simulink model "lab1_1"  (R2021b)
settings: Solver=VariableStepAuto  StartTime=0.0  StopTime=30  RelTol=10e-10  AbsTol=10e-10
values from neighbouring files (symbols this model uses):
  den = cell2mat(den)    [lab1.m]
  den1 = cell2mat(den1)    [lab1.m]
  num = cell2mat(num)    [lab1.m]
  num1 = cell2mat(num1)    [lab1.m]
settings Model: Creator=zhangshaoyang  LastModifiedBy=zhangshaoyang

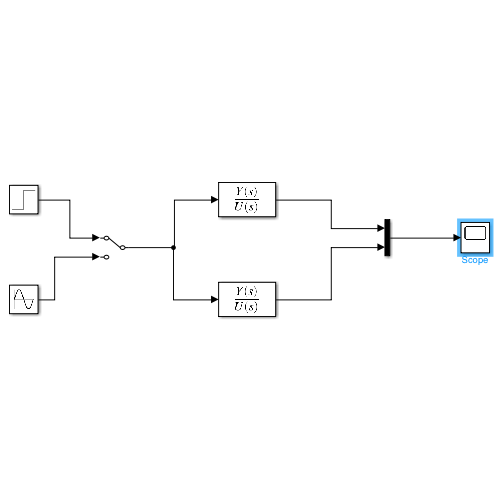
[thumbnail: Simulink's stored preview of the top-level diagram]
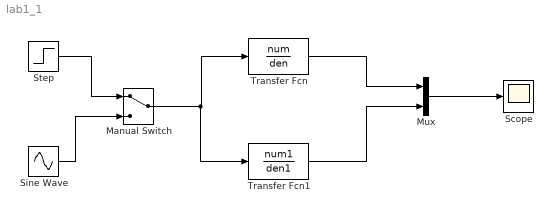
== system lab1_1 ==
  Manual Switch : ManualSwitch
  Mux : Mux  Inputs=2
  Scope : Scope
  Sine Wave : Sin  SampleTime=0
  Step : Step  SampleTime=0
  Transfer Fcn : TransferFcn  Numerator=num  Denominator=den
  Transfer Fcn1 : TransferFcn  Numerator=num1  Denominator=den1
  wires:
  Step/1 -> Manual Switch/1
  Sine Wave/1 -> Manual Switch/2
  Manual Switch/1 -> Transfer Fcn1/1, Transfer Fcn/1
  Transfer Fcn/1 -> Mux/1
  Transfer Fcn1/1 -> Mux/2
  Mux/1 -> Scope/1
